simulink model "simlink_files"  (R2017a)
settings: Solver=VariableStepAuto  StartTime=0.0  StopTime=150  RelTol=1e-3
libraries: cstblocks x1
settings Model: Creator=Night Fury  LastModifiedBy=Havoc

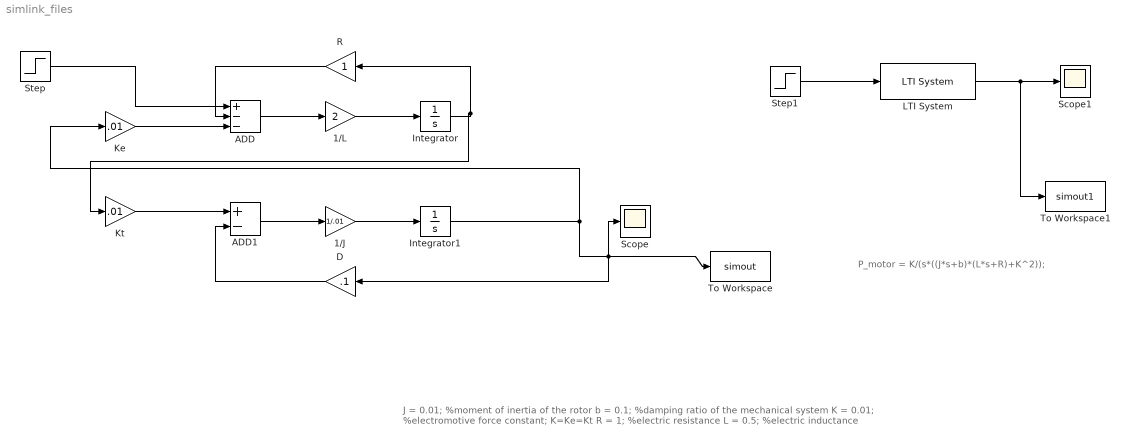
== system simlink_files ==
  note: P_motor = K/(s*((J*s+b)*(L*s+R)+K^2));
  note: J = 0.01; %moment of inertia of the rotor
      | b = 0.1; %damping ratio of the mechanical system
      | K = 0.01; %electromotive force constant; K=Ke=Kt
      | R = 1; %electric resistance L = 0.5; %electric inductance
  1/J : Gain  Gain=1/.01
  1/L : Gain  Gain=2
  ADD : Sum  Inputs=+--
  ADD1 : Sum  Inputs=+-
  D : Gain  Gain=.1
  Integrator : Integrator
  Integrator1 : Integrator
  Ke : Gain  Gain=.01
  Kt : Gain  Gain=.01
  LTI System : cstblocks/LTI System  sys=tf([0 .01],[.5*.01 1*.01+.1*.5 .01*.01+1*.1])  IC=[]
  R : Gain
  Scope : Scope
  Scope1 : Scope
  Step : Step  Time=0  SampleTime=0
  Step1 : Step  Time=0  SampleTime=0
  To Workspace : ToWorkspace  VariableName=simout  SampleTime=-1
      settings: Save2DSignal=2-D array (concatenate along first dimension)
  To Workspace1 : ToWorkspace  VariableName=simout1  SampleTime=-1
      settings: Save2DSignal=2-D array (concatenate along first dimension)
  wires:
  LTI System/1 -> To Workspace1/1, Scope1/1
  Step1/1 -> LTI System/1
  Kt/1 -> ADD1/1
  ADD1/1 -> 1/J/1
  1/L/1 -> Integrator/1
  R/1 -> ADD/2
  1/J/1 -> Integrator1/1
  ADD/1 -> 1/L/1
  Integrator/1 -> Kt/1, R/1
  Step/1 -> ADD/1
  Ke/1 -> ADD/3
  Integrator1/1 -> To Workspace/1, D/1, Scope/1, Ke/1
  D/1 -> ADD1/2
